simulink model "CH22_3D"  (Simulink 10.1)
settings: Solver=ode45  StartTime=0.0  StopTime=20  RelTol=1e-3  EnableMultiTasking=on
libraries: commfilt2 x2, commrandsrc2 x2, commutil2 x2, simulink x1
settings Model: Creator=my2  LastModifiedBy=IT
settings DataIOCC: LimitDataPoints=on  SignalLoggingSaveFormat=ModelDataLogs
settings DebuggingCC: SolverPrmCheckMsg=warning  MultiTaskDSMMsg=warning  MultiTaskCondExecSysMsg=none  FcnCallInpInsideContextMsg=warning

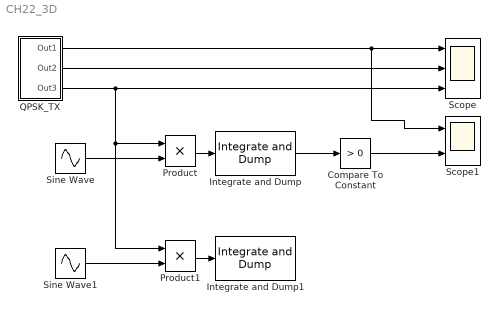
== system CH22_3D ==
  Compare To Constant : simulink/Logic and Bit Operations/Compare To Constant  relop=>  const=0  OutDataTypeStr=boolean
  Integrate and Dump : commfilt2/Integrate and Dump  obssamples=8  offsetsamples=0  nodump=off  roundingMode=Floor  overflowMode=off  outputDataTypeStr=Inherit: Same as accumulator  outputLastDataTypeStr=Inherit: Same as accumulator
  Integrate and Dump1 : commfilt2/Integrate and Dump  obssamples=8  offsetsamples=0  nodump=off  roundingMode=Floor  overflowMode=off  outputDataTypeStr=Inherit: Same as accumulator  outputLastDataTypeStr=Inherit: Same as accumulator
  Product : Product
  Product1 : Product
  QPSK_TX : Subsystem
  Scope : Scope  NumInputPorts=3
  Scope1 : Scope  NumInputPorts=2
  Sine Wave : Sin  SampleTime=1/256
  Sine Wave1 : Sin  SampleTime=1/256
  wires:
  QPSK_TX/1(Out1) -> Scope1/1, Scope/1
  QPSK_TX/2(Out2) -> Scope/2
  Sine Wave/1 -> Product/2
  Product/1 -> Integrate and Dump/1
  QPSK_TX/3(Out3) -> Scope/3, Product/1, Product1/1
  Sine Wave1/1 -> Product1/2
  Product1/1 -> Integrate and Dump1/1
  Integrate and Dump/1 -> Compare To Constant/1
  Compare To Constant/1 -> Scope1/2

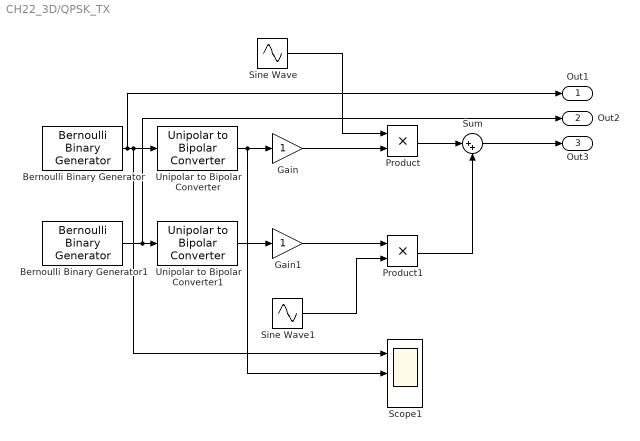
== system CH22_3D/QPSK_TX ==
  Bernoulli Binary Generator : commrandsrc2/Bernoulli Binary Generator  SystemSampleTime=-1  P=0.5  seed=20301181  Ts=1  frameBased=off  sampPerFrame=1  orient=off  outDataType=boolean
      settings: SourceProductBaseCode=CM
  Bernoulli Binary Generator1 : commrandsrc2/Bernoulli Binary Generator  SystemSampleTime=-1  P=0.5  seed=7  Ts=1  frameBased=off  sampPerFrame=1  orient=off  outDataType=boolean
      settings: SourceProductBaseCode=CM
  Gain : Gain
  Gain1 : Gain
  Product : Product
  Product1 : Product
  Scope1 : Scope  NumInputPorts=3
  Sine Wave : Sin  SampleTime=1/256
  Sine Wave1 : Sin  SampleTime=1/256
  Sum : Sum  Inputs=|++
  Unipolar to Bipolar Converter : commutil2/Unipolar to Bipolar Converter  SystemSampleTime=-1  M=2  polarity=Positive  dataType=Inherit via internal rule
  Unipolar to Bipolar Converter1 : commutil2/Unipolar to Bipolar Converter  SystemSampleTime=-1  M=2  polarity=Positive  dataType=Inherit via internal rule
  Out1 : Outport
  Out2 : Outport  Port=2
  Out3 : Outport  Port=3
  wires:
  Sum/1 -> Out3/1
  Unipolar to Bipolar Converter/1 -> Scope1/2, Gain/1
  Sine Wave1/1 -> Product1/2
  Gain1/1 -> Product1/1
  Sine Wave/1 -> Product/1
  Bernoulli Binary Generator/1 -> Out1/1, Scope1/1, Unipolar to Bipolar Converter/1
  Product/1 -> Sum/1
  Product1/1 -> Sum/2
  Unipolar to Bipolar Converter1/1 -> Gain1/1
  Bernoulli Binary Generator1/1 -> Out2/1, Unipolar to Bipolar Converter1/1
  Gain/1 -> Product/2
